simulink model "randamentul_pompei"  (R2022b)
settings: Solver=VariableStepAuto  StartTime=0.0  StopTime=10.0  RelTol=1e-3
values from neighbouring files (symbols this model uses):
  keta = 8*(10^-5)    (= 8e-05)    [date_indrumator.m]    (also in proiect.m)
settings Model: Creator=Ruxandra  LastModifiedBy=Ruxandra

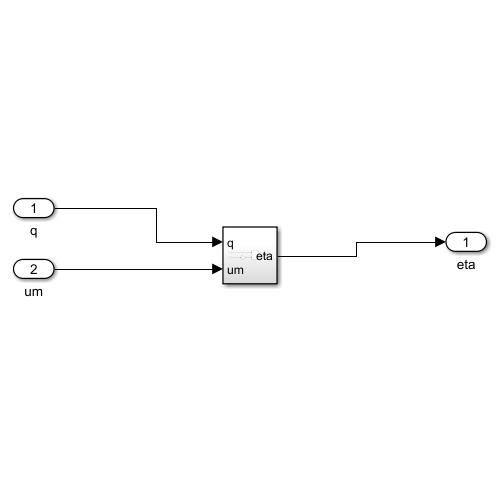
[thumbnail: Simulink's stored preview of the top-level diagram]
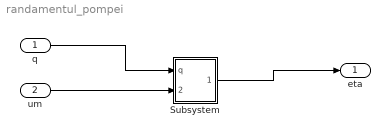
== system randamentul_pompei ==
  q : Inport
  um : Inport  Port=2
  Subsystem : Subsystem
  eta : Outport
  wires:
  q/1 -> Subsystem/1(q)
  um/1 -> Subsystem/2(um)
  Subsystem/1(eta) -> eta/1

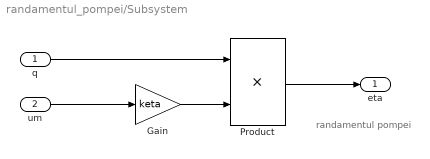
== system randamentul_pompei/Subsystem ==
  note: randamentul pompei
  q : Inport
  um : Inport  Port=2
  Gain : Gain  Gain=keta
  Product : Product
  eta : Outport
  wires:
  um/1 -> Gain/1
  Product/1 -> eta/1
  q/1 -> Product/1
  Gain/1 -> Product/2
